simulink model "Luenberger_Observer"  (R2025a)
settings: Solver=VariableStepAuto  StartTime=0.0  StopTime=10.0  RelTol=1e-3
settings Model: Creator=xing2  LastModifiedBy=xing2

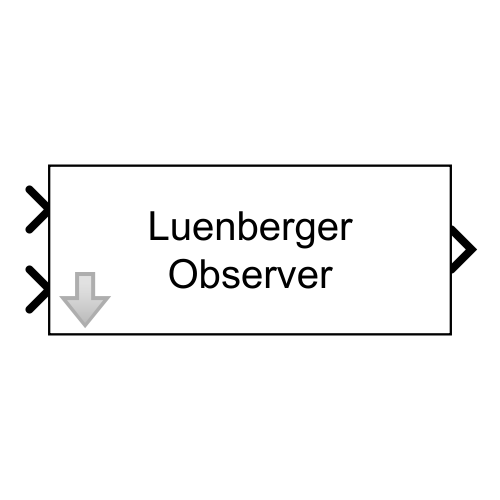
[thumbnail: Simulink's stored preview of the top-level diagram]
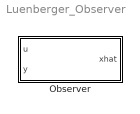
== system Luenberger_Observer ==
  Observer : Subsystem  mask{A_obs=[0 1;-10 -0.5], B_aug=[0 5;1 10], C_obs=[1 0;0 1], D_aug=[0 0;0 0], x0=[0;0]}
      mask prompts: A_obs "A matrix"; B_aug "B_aug=[B L]"; C_obs "C matrix"; D_aug "D matrix"
      mask help: Luenberger Observer: dxhat=A*xhat+[B,L]*[u;y]. B_aug=[B, L]
      mask Display: disp('Luenberger\nObserver');

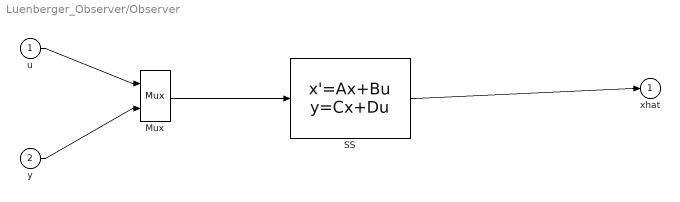
== system Luenberger_Observer/Observer ==
  u : Inport
  y : Inport  Port=2
  Mux : Mux  Inputs=2
  SS : StateSpace  A=A_obs  B=B_aug  C=C_obs  D=D_aug  InitialCondition=x0
  xhat : Outport
  wires:
  u/1 -> Mux/1
  y/1 -> Mux/2
  Mux/1 -> SS/1
  SS/1 -> xhat/1
